simulink model "ConnectingWetElectrodes"  (R2020b)
settings: Solver=VariableStepAuto  StartTime=0.0  StopTime=10  RelTol=1e-3
libraries: fl_lib x28, nesl_utility x4, simulink x1
settings Model: Creator=Miodrag Bolic  LastModifiedBy=Miodrag Bolic

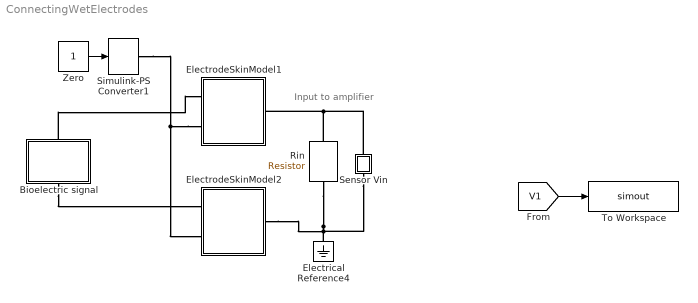
== system ConnectingWetElectrodes ==
  note: Input to amplifier
  Bioelectric signal : Subsystem
      mask Display: image('ECGPicture.png'); % Use "Edit Image" on toolstrip to change.
  Electrical Reference4 : fl_lib/Electrical/Electrical Elements/Electrical Reference
  ElectrodeSkinModel1 : Subsystem
  ElectrodeSkinModel2 : Subsystem
  Rin : fl_lib/Electrical/Electrical Elements/Resistor  R=20 MOhm  i_specify=off  i_priority=None  i=0 A  i_nominal_specify=off  i_nominal_unit=A  i_nominal_value=1  v_specify=off  v_priority=None  v=0 V  v_nominal_specify=off  v_nominal_unit=V  v_nominal_value=1
  Sensor Vin : Subsystem
      mask Display: disp('v')
  Simulink-PS Converter1 : nesl_utility/Simulink-PS Converter  PhysicalDomain=network_engine_domain  SubClassName=ps_input  LeftPortType=input  RightPortType=output  PseudoPeriodic=off  Frequencies=[]  NoiseDistribution=none  NoiseParameters=[]  Unit=1  AffineConversion=off  FilteringAndDerivatives=zero  SimscapeFilterOrder=1  InputFilterTimeConstant=0.001  UdotUserProvided=1
  To Workspace : ToWorkspace  VariableName=simout  SaveFormat=Timeseries  SampleTime=-1
  Zero : Constant  OutDataTypeStr=Inherit: Inherit via back propagation
  wires:
  Zero/1 -> Simulink-PS Converter1/1
  [V1] -> To Workspace/1
  connections:
  ElectrodeSkinModel1/LConn2 -- ElectrodeSkinModel2/LConn2 -- Simulink-PS Converter1/RConn1
  Bioelectric signal/LConn1 -- ElectrodeSkinModel1/LConn1
  Bioelectric signal/RConn1 -- ElectrodeSkinModel2/LConn1
  Rin/LConn1 -- Sensor Vin/RConn1 -- ElectrodeSkinModel1/RConn1
  Rin/RConn1 -- ElectrodeSkinModel2/RConn1 -- Sensor Vin/LConn1 -- Electrical Reference4/LConn1

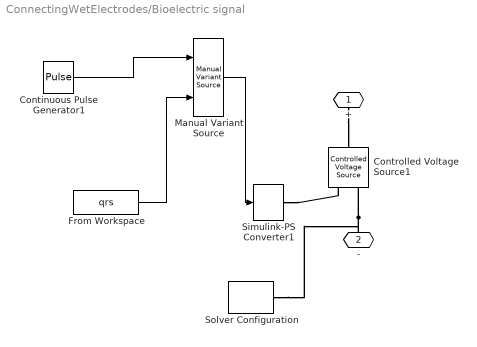
== system ConnectingWetElectrodes/Bioelectric signal ==
  Continuous Pulse Generator1 : DiscretePulseGenerator  PulseType=Time based  Amplitude=0.001  Period=1  PulseWidth=10
  Controlled Voltage Source1 : fl_lib/Electrical/Electrical Sources/Controlled Voltage Source
  From Workspace : FromWorkspace  VariableName=qrs  SampleTime=0.0001  OutputAfterFinalValue=Setting to zero
  Manual Variant Source : simulink/Signal Routing/Manual Variant Source  NumChoices=2  LabelModeActiveChoice=V_1
  Simulink-PS Converter1 : nesl_utility/Simulink-PS Converter  PhysicalDomain=network_engine_domain  SubClassName=ps_input  LeftPortType=input  RightPortType=output  PseudoPeriodic=off  Frequencies=[]  NoiseDistribution=none  NoiseParameters=[]  Unit=1  AffineConversion=off  FilteringAndDerivatives=zero  SimscapeFilterOrder=1  InputFilterTimeConstant=0.001  UdotUserProvided=1
  Solver Configuration : nesl_utility/Solver Configuration  PhysicalDomain=network_engine_domain  SubClassName=solver  LeftPortType=input  RightPortType=generic  Tones=[]  Harmonics=[]  SimulateNoise=off  Profile=off  UseLocalSampling=off  EnableSwitchedLinearOptims=on  FrequencyDomain=off  UseCCode=off  RelTol=0.001  AbsTol=1e-06  MinStep=1e-09  ToWorkspace=off  RevertToSquareIcSolve=off  NumHomotopyIterations=100  PhasorMode=off  PhasorModeNumHarmonics=1  DoDC=off  ResidualTolerance=1e-20  UseLocalSolver=on  LocalSolverChoice=NE_PARTITIONING_ADVANCER  LocalSolverSampleTime=0.0001  DoFixedCost=on  MaxNonlinIter=3  MaxModeIter=2  ComputeImpulses=on  ImpulseIterations=2  LinearAlgebra=auto  EquationFormulation=NE_TIME_EF  DelaysMemoryBudget=1024  AutomaticFiltering=on  FilteringTimeConstant=0.001  PartitionStorageMethod=EXHAUSTIVE  PartitionMemoryBudget=1024  PartitionMethod=ROBUST
  + : PMIOPort  Side=Left
  - : PMIOPort  Port=2  Side=Right
  wires:
  From Workspace/1 -> Manual Variant Source/2
  Manual Variant Source/1 -> Simulink-PS Converter1/1
  Continuous Pulse Generator1/1 -> Manual Variant Source/1
  connections:
  Simulink-PS Converter1/RConn1 -- Controlled Voltage Source1/RConn1
  +/RConn1 -- Controlled Voltage Source1/LConn1
  -/RConn1 -- Solver Configuration/RConn1 -- Controlled Voltage Source1/RConn2

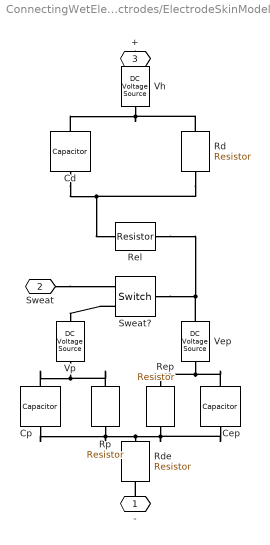
== system ConnectingWetElectrodes/ElectrodeSkinModel1 ==
  Cd : fl_lib/Electrical/Electrical Elements/Capacitor  c=1 nF  r=1e-6 Ohm  g=0 1/Ohm  i_specify=off  i_priority=None  i=0 A  i_nominal_specify=off  i_nominal_unit=A  i_nominal_value=1  v_specify=off  v_priority=None  v=0 V  v_nominal_specify=off  v_nominal_unit=V  v_nominal_value=1  vc_specify=on  vc_priority=High  vc=0 V  vc_nominal_specify=off  vc_nominal_unit=V  vc_nominal_value=1
  Cep : fl_lib/Electrical/Electrical Elements/Capacitor  c=20 nF  r=1e-6 Ohm  g=0 1/Ohm  i_specify=off  i_priority=None  i=0 A  i_nominal_specify=off  i_nominal_unit=A  i_nominal_value=1  v_specify=off  v_priority=None  v=0 V  v_nominal_specify=off  v_nominal_unit=V  v_nominal_value=1  vc_specify=on  vc_priority=High  vc=0 V  vc_nominal_specify=off  vc_nominal_unit=V  vc_nominal_value=1
  Cp : fl_lib/Electrical/Electrical Elements/Capacitor  c=1 pF  r=1e-6 Ohm  g=0 1/Ohm  i_specify=off  i_priority=None  i=0 A  i_nominal_specify=off  i_nominal_unit=A  i_nominal_value=1  v_specify=off  v_priority=None  v=0 V  v_nominal_specify=off  v_nominal_unit=V  v_nominal_value=1  vc_specify=on  vc_priority=High  vc=0 V  vc_nominal_specify=off  vc_nominal_unit=V  vc_nominal_value=1
  Rd : fl_lib/Electrical/Electrical Elements/Resistor  R=5 kOhm  i_specify=off  i_priority=None  i=0 A  i_nominal_specify=off  i_nominal_unit=A  i_nominal_value=1  v_specify=off  v_priority=None  v=0 V  v_nominal_specify=off  v_nominal_unit=V  v_nominal_value=1
  Rde : fl_lib/Electrical/Electrical Elements/Resistor  R=1 kOhm  i_specify=off  i_priority=None  i=0 A  i_nominal_specify=off  i_nominal_unit=A  i_nominal_value=1  v_specify=off  v_priority=None  v=0 V  v_nominal_specify=off  v_nominal_unit=V  v_nominal_value=1
  Rel : fl_lib/Electrical/Electrical Elements/Resistor  R=500 kOhm  i_specify=off  i_priority=None  i=0 A  i_nominal_specify=off  i_nominal_unit=A  i_nominal_value=1  v_specify=off  v_priority=None  v=0 V  v_nominal_specify=off  v_nominal_unit=V  v_nominal_value=1
  Rep : fl_lib/Electrical/Electrical Elements/Resistor  R=500 kOhm  i_specify=off  i_priority=None  i=0 A  i_nominal_specify=off  i_nominal_unit=A  i_nominal_value=1  v_specify=off  v_priority=None  v=0 V  v_nominal_specify=off  v_nominal_unit=V  v_nominal_value=1
  Rp : fl_lib/Electrical/Electrical Elements/Resistor  R=100 Ohm  i_specify=off  i_priority=None  i=0 A  i_nominal_specify=off  i_nominal_unit=A  i_nominal_value=1  v_specify=off  v_priority=None  v=0 V  v_nominal_specify=off  v_nominal_unit=V  v_nominal_value=1
  Sweat? : fl_lib/Electrical/Electrical Elements/Switch  R_closed=0.01 Ohm  G_open=1e-8 1/Ohm  Threshold=0.5  i_specify=off  i_priority=None  i=0 A  i_nominal_specify=off  i_nominal_unit=A  i_nominal_value=1  v_specify=off  v_priority=None  v=0 V  v_nominal_specify=off  v_nominal_unit=V  v_nominal_value=1
  Vep : fl_lib/Electrical/Electrical Sources/DC Voltage Source  v0=20 mV
  Vh : fl_lib/Electrical/Electrical Sources/DC Voltage Source  v0=230 mV
  Vp : fl_lib/Electrical/Electrical Sources/DC Voltage Source  v0=5 mV
  - : PMIOPort  Side=Left
  Sweat : PMIOPort  Port=2  Side=Left
  + : PMIOPort  Port=3  Side=Right
  connections:
  Vp/RConn1 -- Rp/RConn1 -- Cp/RConn1
  Vh/LConn1 -- +/RConn1
  Sweat/RConn1 -- Sweat?/RConn1
  Sweat?/RConn2 -- Vp/LConn1
  Vh/RConn1 -- Rd/RConn1 -- Cd/RConn1
  Cd/LConn1 -- Rd/LConn1 -- Rel/RConn1
  Cep/RConn1 -- Vep/RConn1 -- Rep/RConn1
  Sweat?/LConn1 -- Rel/LConn1 -- Vep/LConn1
  Rp/LConn1 -- Cp/LConn1 -- Cep/LConn1 -- Rep/LConn1 -- Rde/LConn1
  -/RConn1 -- Rde/RConn1

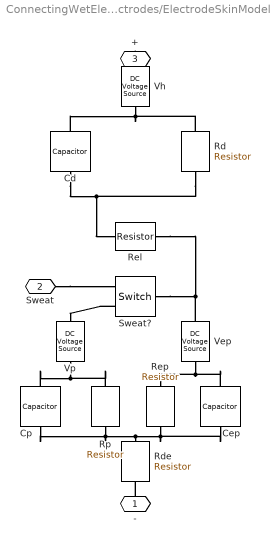
== system ConnectingWetElectrodes/ElectrodeSkinModel2 ==
  Cd : fl_lib/Electrical/Electrical Elements/Capacitor  c=1 nF  r=1e-6 Ohm  g=0 1/Ohm  i_specify=off  i_priority=None  i=0 A  i_nominal_specify=off  i_nominal_unit=A  i_nominal_value=1  v_specify=off  v_priority=None  v=0 V  v_nominal_specify=off  v_nominal_unit=V  v_nominal_value=1  vc_specify=on  vc_priority=High  vc=0 V  vc_nominal_specify=off  vc_nominal_unit=V  vc_nominal_value=1
  Cep : fl_lib/Electrical/Electrical Elements/Capacitor  c=20 nF  r=1e-6 Ohm  g=0 1/Ohm  i_specify=off  i_priority=None  i=0 A  i_nominal_specify=off  i_nominal_unit=A  i_nominal_value=1  v_specify=off  v_priority=None  v=0 V  v_nominal_specify=off  v_nominal_unit=V  v_nominal_value=1  vc_specify=on  vc_priority=High  vc=0 V  vc_nominal_specify=off  vc_nominal_unit=V  vc_nominal_value=1
  Cp : fl_lib/Electrical/Electrical Elements/Capacitor  c=1 pF  r=1e-6 Ohm  g=0 1/Ohm  i_specify=off  i_priority=None  i=0 A  i_nominal_specify=off  i_nominal_unit=A  i_nominal_value=1  v_specify=off  v_priority=None  v=0 V  v_nominal_specify=off  v_nominal_unit=V  v_nominal_value=1  vc_specify=on  vc_priority=High  vc=0 V  vc_nominal_specify=off  vc_nominal_unit=V  vc_nominal_value=1
  Rd : fl_lib/Electrical/Electrical Elements/Resistor  R=5 kOhm  i_specify=off  i_priority=None  i=0 A  i_nominal_specify=off  i_nominal_unit=A  i_nominal_value=1  v_specify=off  v_priority=None  v=0 V  v_nominal_specify=off  v_nominal_unit=V  v_nominal_value=1
  Rde : fl_lib/Electrical/Electrical Elements/Resistor  R=1 kOhm  i_specify=off  i_priority=None  i=0 A  i_nominal_specify=off  i_nominal_unit=A  i_nominal_value=1  v_specify=off  v_priority=None  v=0 V  v_nominal_specify=off  v_nominal_unit=V  v_nominal_value=1
  Rel : fl_lib/Electrical/Electrical Elements/Resistor  R=500 kOhm  i_specify=off  i_priority=None  i=0 A  i_nominal_specify=off  i_nominal_unit=A  i_nominal_value=1  v_specify=off  v_priority=None  v=0 V  v_nominal_specify=off  v_nominal_unit=V  v_nominal_value=1
  Rep : fl_lib/Electrical/Electrical Elements/Resistor  R=500 kOhm  i_specify=off  i_priority=None  i=0 A  i_nominal_specify=off  i_nominal_unit=A  i_nominal_value=1  v_specify=off  v_priority=None  v=0 V  v_nominal_specify=off  v_nominal_unit=V  v_nominal_value=1
  Rp : fl_lib/Electrical/Electrical Elements/Resistor  R=100 Ohm  i_specify=off  i_priority=None  i=0 A  i_nominal_specify=off  i_nominal_unit=A  i_nominal_value=1  v_specify=off  v_priority=None  v=0 V  v_nominal_specify=off  v_nominal_unit=V  v_nominal_value=1
  Sweat? : fl_lib/Electrical/Electrical Elements/Switch  R_closed=0.01 Ohm  G_open=1e-8 1/Ohm  Threshold=0.5  i_specify=off  i_priority=None  i=0 A  i_nominal_specify=off  i_nominal_unit=A  i_nominal_value=1  v_specify=off  v_priority=None  v=0 V  v_nominal_specify=off  v_nominal_unit=V  v_nominal_value=1
  Vep : fl_lib/Electrical/Electrical Sources/DC Voltage Source  v0=20 mV
  Vh : fl_lib/Electrical/Electrical Sources/DC Voltage Source  v0=230 mV
  Vp : fl_lib/Electrical/Electrical Sources/DC Voltage Source  v0=5 mV
  - : PMIOPort  Side=Left
  Sweat : PMIOPort  Port=2  Side=Left
  + : PMIOPort  Port=3  Side=Right
  connections:
  Vp/RConn1 -- Rp/RConn1 -- Cp/RConn1
  Vh/LConn1 -- +/RConn1
  Sweat/RConn1 -- Sweat?/RConn1
  Sweat?/RConn2 -- Vp/LConn1
  Vh/RConn1 -- Rd/RConn1 -- Cd/RConn1
  Cd/LConn1 -- Rd/LConn1 -- Rel/RConn1
  Cep/RConn1 -- Vep/RConn1 -- Rep/RConn1
  Sweat?/LConn1 -- Rel/LConn1 -- Vep/LConn1
  Rp/LConn1 -- Cp/LConn1 -- Cep/LConn1 -- Rep/LConn1 -- Rde/LConn1
  -/RConn1 -- Rde/RConn1

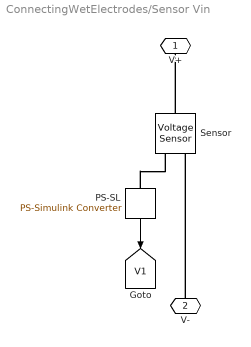
== system ConnectingWetElectrodes/Sensor Vin ==
  PS-SL : nesl_utility/PS-Simulink Converter  PhysicalDomain=network_engine_domain  SubClassName=ps_output  LeftPortType=input  RightPortType=output  PseudoPeriodic=off  Frequencies=[]  Unit=1  AffineConversion=off
  Sensor : fl_lib/Electrical/Electrical Sensors/Voltage Sensor
      settings: SourceProductName=Foundation Library
  V+ : PMIOPort  Side=Right
  V- : PMIOPort  Port=2  Side=Left
  tag scope: V1=global
  wires:
  PS-SL/1 -> [V1]
  connections:
  PS-SL/LConn1 -- Sensor/RConn1
  Sensor/LConn1 -- V+/RConn1
  V-/RConn1 -- Sensor/RConn2
